simulink model "test_q"  (R2014a)
settings: Solver=ode3  StartTime=0.0  StopTime=100  RelTol=1e-3
settings Model: Creator=Iseberg  LastModifiedBy=Iseberg

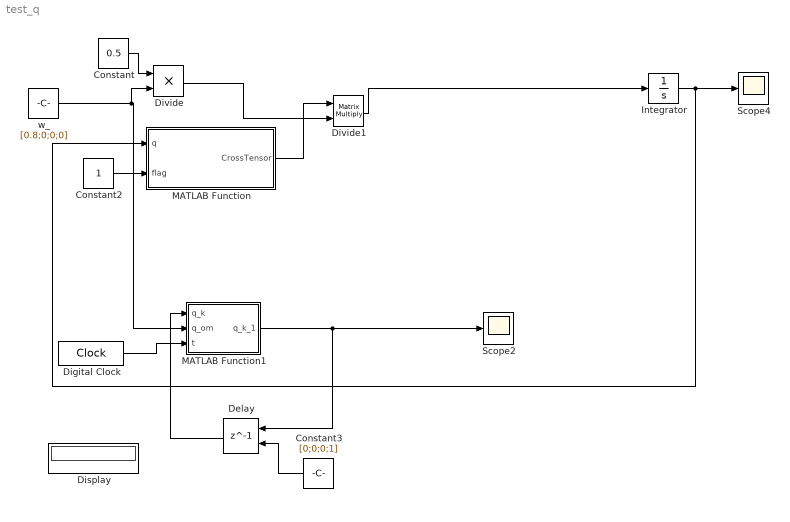
== system test_q ==
  Constant : Constant  Value=0.5
  Constant2 : Constant
  Constant3 : Constant  Value=[0;0;0;1]
  Delay : Delay  DelayLength=1  InitialConditionSource=Input port  InitialCondition=0
      settings: InputPortMap=u0,p4
  Digital Clock : DigitalClock  SampleTime=-1
  Display : Display
  Divide : Product  Inputs=**
  Divide1 : Product  Inputs=**  Multiplication=Matrix(*)
  Integrator : Integrator  InitialCondition=[0;0;0;1]
  MATLAB Function : MATLAB Function  TreatAsAtomicUnit=on
  MATLAB Function1 : MATLAB Function  TreatAsAtomicUnit=on
  Scope2 : Scope
      settings: SaveName=ScopeData2
  Scope4 : Scope
      settings: SaveName=ScopeData4
  w_ : Constant  Value=[0.8;0;0;0]
  wires:
  Constant/1 -> Divide/1
  w_/1 -> MATLAB Function1/2(q_om), Divide/2
  Divide1/1 -> Integrator/1
  Constant2/1 -> MATLAB Function/2(flag)
  MATLAB Function/1(CrossTensor) -> Divide1/1
  Divide/1 -> Divide1/2
  MATLAB Function1/1(q_k_1) -> Delay/1, Scope2/1
  Digital Clock/1 -> MATLAB Function1/3(t)
  Integrator/1 -> Scope4/1, MATLAB Function/1(q)
  Constant3/1 -> Delay/2
  Delay/1 -> MATLAB Function1/1(q_k)

== matlab function test_q/MATLAB Function1 ==
  data: q_k input; q_k_1 output; q_om input; t input
function q_k_1 = fcn(q_k,q_om,t)
%#codegen
    q_k_1 = fn_CreateNominal_q_test(q_om,0.01,0,q_k);
    
    %q = q/norm(q);
end

== matlab function test_q/MATLAB Function ==
  data: q input; CrossTensor output; flag input
%Inputs: q: quaternion vector
%        flag:0-cross;1-star
function CrossTensor  = fn_CrossTensor(q,flag)
    CrossTensor = zeros(4,4);
    q_v = q(1:3);
    q_0 = q(4);    
    cross_q_v = fn_VectorToSkewSymmetricTensor(q_v);
    switch (flag)
        case 0
            CrossTensor = [-cross_q_v + q_0*eye(3,3), q_v;-q_v',q_0];
        case 1
            CrossTensor = [cross_q_v + q_0*eye(3,3), q_v;-q_v',q_0];
        otherwise
            
    end
end
